simulink model "Lidar_System_July10_lidarCam"  (Simulink 7.3)
settings: Solver=FixedStepDiscrete  StartTime=0.0  StopTime=inf  FixedStep=0.1  MaxStep=0.2  RelTol=1e-3
undefined symbols (not defined in the file): strel
libraries: dspmtrx3 x9, dspstat3 x4, simulink x3, vipstatistics x2, vipgeotforms x1, vipmorphops x1
(part 5 of 7)

== matlab function Enabled Subsystem1/Data Save Interpolation and Bayes/Template Matching Subsystem/Detection/Detection ==
  data: cruciform input double; bbox_out output double; circle input double; triangle input double; whitePixCount input double; threshold input double; V_mask input double; bbox_in input double; label input double; rtnRatioDiff output double
function [bbox_out,rtnRatioDiff]= detection(cruciform,circle,triangle,...
    whitePixCount,threshold,V_mask,bbox_in,label)

% Written by Edward Zhu on 5/14/14
% Last Edited by Anderson Lebbad on 7/10/14 - adapted for r2009a

% Inputs
% tempID:       Number corresponding to one of the templates (cruciform: 1,
%               circle: 2, triangle: 3)
% cruciform:    19*19 template of cruciform
% circle:       19*19 template of circle
% triangle:     19*19 template of triangle
% whitePixCount:Number of white pixels in each of the templates
% V_mask:       V channel binary mask
% bbox_in:      Bounding boxes as found by blob analysis
% label:        Label matrix as found by blob analysis

% Outputs
% bbox_out:     Bounding box of matched symbol
% symFound:     Status of matching (found: 1, not found: 0)

% Define frame and template size
templates = zeros(19,19,3);
templates(:,:,1) = cruciform;
templates(:,:,2) = circle;
templates(:,:,3) = triangle;

imgRows = size(label,1);
imgCols = size(label,2);
tempRows = size(templates,1);
tempCols = size(templates,2);
numBBox = size(bbox_in,2);

% Initialize scaled image and output bbox matrices
V_scaled = zeros(tempRows,tempCols);
bbox_out = uint32(zeros(4,numBBox));
rtnRatioDiff = ones(numBBox,1);

bestRatioDiff = single(1);

for i = 1:numBBox
    shapeDiff = abs(1-bbox_in(4,i)/bbox_in(3,i));
    if bbox_in(4,i) >= tempCols && bbox_in(3,i) >= tempRows && shapeDiff < 0.5
        % Set up arrays for the start and end rows and columns for bbox
        % matching
        
        similarity = zeros(1,3);
        ratioDiff = zeros(1,3);
        
        rowStep = floor(bbox_in(3,i) / tempRows);
        colStep = floor(bbox_in(4,i) / tempCols);
        
        startRowList = zeros(1,3);
        startRowList(2) = bbox_in(1,i)+1;
        startRowList(1) = max(1, startRowList(2) - rowStep);
        startRowList(3) = min(imgRows, startRowList(2) + rowStep);
        
        endRowList = zeros(1,3);
        endRowList(2) = bbox_in(1,i)+1 + bbox_in(3,i);
        endRowList(1) = max(1, endRowList(2) - rowStep);
        endRowList(3) = min(imgRows, endRowList(2) + rowStep);
        
        startColList = zeros(1,3);
        startColList(2) = bbox_in(2,i)+1;
        startColList(1) = max(1, startColList(2) - colStep);
        startColList(3) = min(imgCols, startColList(2) + colStep);
        
        endColList = zeros(1,3);
        endColList(2) = bbox_in(2,i)+1 + bbox_in(i,3);
        endColList(1) = max(1, endColList(2) - colStep);
        endColList(3) = min(imgCols, endColList(2) + colStep);
        
        % Scale down image in bbox to size of template (18*18 px)
        for startRow = startRowList
            for endRow = endRowList
                rowScaleStep = floor((endRow - startRow) / tempRows);
                
                for startCol = startColList
                    for endCol = endColList
                        colScaleStep = floor((endCol - startCol) / tempCols);
                        
                        captureRow = startRow;
                        for row = 1:tempRows
                            captureCol = startCol;
                            for col = 1:tempCols
                                V_scaled(row,col) = V_mask(captureRow,captureCol);
                                for tempID = 1:3
                                    similarity(tempID) = similarity(tempID) + templates(row,col,tempID) * (V_mask(captureRow,captureCol)*(-1) + 1);
                                end
                                captureCol = captureCol + colScaleStep;                        
                            end
                            captureRow = captureRow + rowScaleStep;
                        end                  
                        
                        for tempID = 1:3   
                            ratioDiff(tempID) = abs(1 - single(similarity(tempID)) / single(whitePixCount(tempID))); 
                        end
                        
                        if min(ratioDiff) < bestRatioDiff
                            bestRatioDiff = single(min(ratioDiff));
                        end
                    end
                end
            end
        end
        
        % Output valid bounding boxes
        if bestRatioDiff < threshold
            bbox_out(:,i) = bbox_in(:,i);
            rtnRatioDiff(i) = bestRatioDiff;
        end
    end
end

== matlab function Enabled Subsystem1/Data Save Interpolation and Bayes/Raster to UV ==
  data: uv_d output double; dist_im input double
function uv_d   = AngleMatch( dist_im )
%Written by Anderson Lebbad on July 8, 2014
%Last Edited:

%This function infers depth locations into a image plane based upon the
%angles as they relate to the field of view of the camera. This works
%decently, but loses accuracy at closer ranges as the spacial translation
%between the video camera and lidar becomes more noticeable

%% Initialize

uv_d = zeros(120,160);

%% Parameters

%Camera field of view to determines indices to match
FoVx = 62;
FoVy = 46;

%Scan angles for lidar gimbal
upAngle = 30;
downAngle = -45;
angleRange = upAngle-downAngle;

%% Operation

% Depth frame, same aspect ratio as image frame, quarter width and height
for i = 1:160
    for j = 1:120
        % Effective coordinate in pixel frame
        u = (i-1)/(160-1)*(640-1)+1;
        v = (j-1)/(120-1)*(480-1)+1;
        
        % Scan angle for pixel location being analyzed in degrees
        scanAngleHoriz = -FoVx/2 + (u-1)*FoVx/(640-1);
        scanAngleVert = FoVy/2 - (v-1)*FoVy/(480-1) + 6;
        
        % Estimate closest scan value for pixel being evaluated
        xCenter = round((67.5+scanAngleHoriz)*(540-1)/135+1);
        yCenter = round((upAngle-scanAngleVert)*(65-1)/(angleRange)+1);
        
        % Assign
        uv_d(j,i) = dist_im(yCenter,xCenter);
    end
end

end

== matlab function Enabled Subsystem1/Data Save Interpolation and Bayes/Template Matching Subsystem/Recognition/Recognition ==
  data: targetTemp input double; cruciform input double; bbox_out output double; circle input double; triangle input double; whitePixCount input double; threshold input double; V_mask input double; bbox_in input double; returnRatioDiff output double
function [bbox_out,returnRatioDiff] = recognition(targetTemp,cruciform,circle,triangle,...
    whitePixCount,threshold,V_mask,bbox_in)

% Written by Edward Zhu on 5/14/14

% Inputs
% tempID:       Number corresponding to one of the templates (cruciform: 1,
%               circle: 2, triangle: 3)
% cruciform:    19*19 template of cruciform
% circle:       19*19 template of circle
% triangle:     19*19 template of triangle
% whitePixCount:Number of white pixels in each of the templates
% V_mask:       V channel binary mask
% bbox_in:      Bounding boxes as found by blob analysis
% label:        Label matrix as found by blob analysis

% Outputs
% bbox_out:     Bounding box of matched symbol
% symFound:     Status of matching (found: 1, not found: 0)

% Define frame and template size
templates = zeros(19,19,3);
templates(:,:,1) = cruciform;
templates(:,:,2) = circle;
templates(:,:,3) = triangle;
templates = 2*(templates-0.5);

tempRows = size(templates,1);
tempCols = size(templates,2);
numBBox = size(bbox_in,2);

% Initialize scaled image and output bbox matrices
V_scaled = zeros(tempRows,tempCols);
bbox_out = uint32(zeros(4,numBBox));

returnRatioDiff = ones(numBBox,1);

for i = 1:numBBox
    if min(bbox_in(:,i)) >= 0
        similarity = 0;
        rowScaleStep = floor(bbox_in(3,i) / tempRows);
        colScaleStep = floor(bbox_in(4,i) / tempCols);
        
        captureRow = bbox_in(1,i)+1;
        for row = 1:tempRows
            captureCol = bbox_in(2,i)+1;
            for col = 1:tempCols
                V_scaled(row,col) = V_mask(captureRow,captureCol);
                similarity = similarity + templates(row,col,targetTemp) * (V_mask(captureRow,captureCol)*(-1) + 1);
                captureCol = captureCol + colScaleStep;
            end
            captureRow = captureRow + rowScaleStep;
        end
        
        ratioDiff = abs(1 - single(similarity) / single(whitePixCount(targetTemp)));
        
        % Output valid bounding box
        if ratioDiff < threshold
            bbox_out(:,i) = bbox_in(:,i);
            returnRatioDiff(i) = ratioDiff;
        end
    end
end

== matlab function Enabled Subsystem1/Data Save Interpolation and Bayes/Template Matching Subsystem/Bay Position ==
  data: xRec input double; bayNumber output double; xDet input double
function bayNumber = bayPosition(xRec,xDet)

symxpos = xRec(1);

if size(xDet,2) == 3
    diff1 = xDet(1) - symxpos;
    diff2 = xDet(2) - symxpos;
    diff3 = xDet(3) - symxpos;
    
    if diff1 == 0
        bayNumber = uint8(1);
    elseif diff2 == 0
        bayNumber = uint8(2);
    elseif diff3 == 0
        bayNumber = uint8(3);
    else
        bayNumber = uint8(0);
    end
    
else
    bayNumber = uint8(0);
end

== matlab function Enabled Subsystem1/Data Save Interpolation and Bayes/Embedded MATLAB Function1 ==
  data: bbox input double; HMean output double; BW input double; uv_d input double; H input double; S input double; V input double; SMean output double; VMean output double; DMean output double; Angle output double
function [HMean, SMean, VMean, DMean, Angle] = bbox_hist(bbox, BW, uv_d, H, S, V)
%This function creates a histogram of the color region of a detected object
%identified in a binary image within a bounding box

%Initialize variables
pixels = 0;
DRunAve = 0;
HRunAve = 0;
SRunAve = 0;
VRunAve = 0;
CDist = 0;
FoV = 62;

%Parse bbox data
left = bbox(2) + 1;
right = left + bbox(4) - 1;
bottom = bbox(1) + 1;
top = bottom + bbox(3) - 1;
Angle = int32((left + bbox(4)/2-320)/320*FoV/2);

%Check to see if valid bbox is found
if left~=-1
    %Scan the detected region of the binary image and generate histograms
    for j=left:right
        for i=bottom:top
            if BW(i,j) == 1
                pixels = pixels + 1;
                DRunAve = ((pixels-1)/pixels)*DRunAve + (1/pixels)*double(uv_d(i,j));
                HRunAve = ((pixels-1)/pixels)*HRunAve + (1/pixels)*double(H(i,j));
                SRunAve = ((pixels-1)/pixels)*SRunAve + (1/pixels)*double(S(i,j));
                VRunAve = ((pixels-1)/pixels)*VRunAve + (1/pixels)*double(V(i,j));
            end
        end
    end
    %CDist = uv_d(left,right);
end

%Means must be integers to use in Bayes Filter
DMean = int32(DRunAve/10);
%DMean = int32(CDist);
HMean = uint8(HRunAve);
SMean = uint8(SRunAve);
VMean = uint8(VRunAve);

end
